simulink model "Regelstrecke_lineare_Zustandsrueckfuehrung"  (R2025a)
settings: Solver=ode15s  StartTime=0.0  StopTime=10
InitFcn:
  | % Definition der Konstanten
  | k  = 1.380649e-23;
  | e  = 1.602176634e-19;
  | T0 = 273.15; % absoluter Nullpunkt in K
  | T_C = 25; % Temperatur in °C
  | UT = k * (T0 + T_C) / e;
  | IS = 1e-8;
  | R  = 1e3;
  | L  = 100e-3;
  | C1 = 100e-9;
  | C2 = 1e-6;
  | 
  | % Werte der Stellgrößen
  | I0 = 10e-3;
  | U0 = 12;
  | 
  | % Berechnung von U2 in der GGL
  | U2_bar = -UT*log(1e8*I0);
  | 
  | % Vorgabe der Eigenwerte
  | eigenvalues = [-200-200i; -200+200i; -500];
  | 
  | % Jacobi-Matrizen an der GGL
  | A = [0 IS/(C1*UT)*exp(-U2_bar/UT) 1/C1;
  |      0 0 1/C2;
  |     -1/L -1/L -R/L];
  | B = [0, 0;
  |      0, -1/C2;
  |      1/L, 0];
  | 
  | % Berechnung der Reglermatrix G
  | G = place(A,B,eigenvalues);
settings Model: Creator=richa  LastModifiedBy=richa

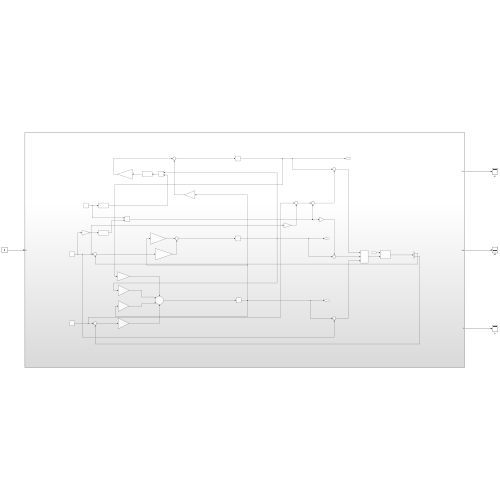
[thumbnail: Simulink's stored preview of the top-level diagram]
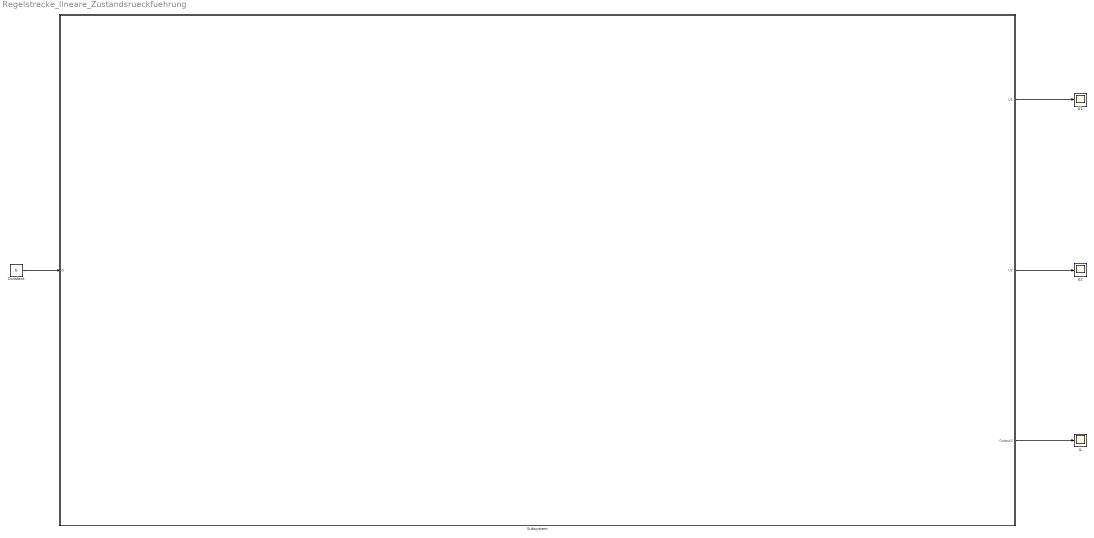
== system Regelstrecke_lineare_Zustandsrueckfuehrung ==
  Constant : Constant  Value=G
  IL : Scope
      settings: ActiveDisplayYMinimum=-0.00074885563020971307  ActiveDisplayYMaximum=0.01042148739337458  DataLoggingVariableName=ScopeData2
  Subsystem : Subsystem
  U1 : Scope
      settings: ActiveDisplayYMinimum=-2.2337880911917134  ActiveDisplayYMaximum=11.108858915218935
  U2 : Scope
      settings: ActiveDisplayYMinimum=-0.762626588701693  ActiveDisplayYMaximum=2.7915785481526711
  wires:
  Subsystem/1(U1) -> U1/1
  Subsystem/2(U2) -> U2/1
  Subsystem/3(Output2) -> IL/1
  Constant/1 -> Subsystem/1("G ")

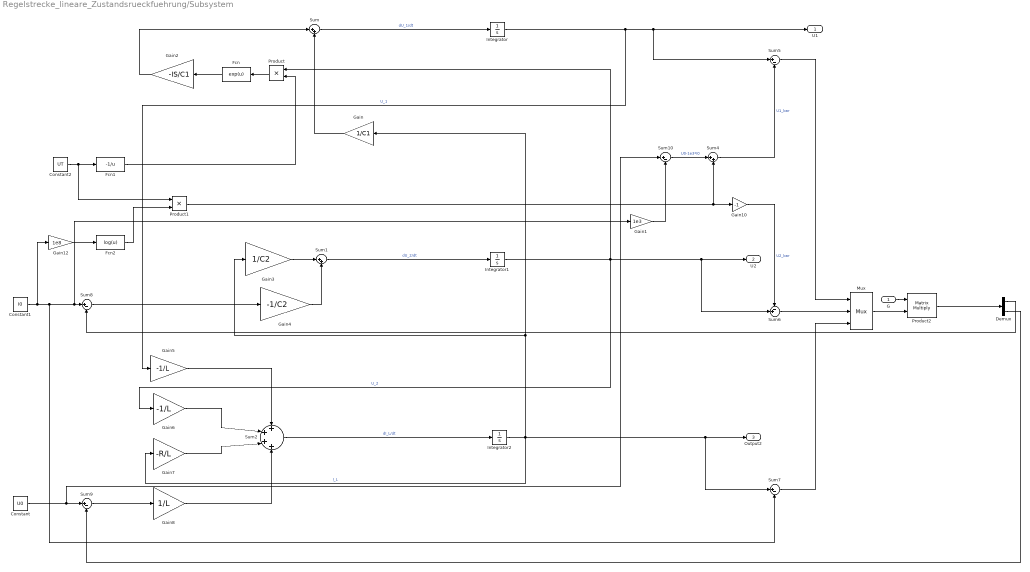
== system Regelstrecke_lineare_Zustandsrueckfuehrung/Subsystem ==
  "G " : Inport
  Constant : Constant  Value=U0
  Constant1 : Constant  Value=I0
  Constant2 : Constant  Value=UT
  Demux : Demux  Outputs=2
  Fcn : Fcn  Expr=exp(u)
  Fcn1 : Fcn  Expr=-1/u
  Fcn2 : Fcn  Expr=log(u)
  Gain : Gain  Gain=1/C1
  Gain1 : Gain  Gain=1e3
  Gain10 : Gain  Gain=-1
  Gain12 : Gain  Gain=1e8
  Gain2 : Gain  Gain=-IS/C1
  Gain3 : Gain  Gain=1/C2
  Gain4 : Gain  Gain=-1/C2
  Gain5 : Gain  Gain=-1/L
  Gain6 : Gain  Gain=-1/L
  Gain7 : Gain  Gain=-R/L
  Gain8 : Gain  Gain=1/L
  Integrator : Integrator
  Integrator1 : Integrator
  Integrator2 : Integrator
  Mux : Mux  Inputs=3
  Product : Product
  Product1 : Product
  Product2 : Product  Multiplication=Matrix(*)
  Sum : Sum  Inputs=|++
  Sum1 : Sum  Inputs=|++
  Sum{5,7..10} (5 alike) : Sum  Inputs=|+-
  Sum2 : Sum  Inputs=++++
  Sum4 : Sum  Inputs=|++
  Sum6 : Sum  Inputs=-+|
  U1 : Outport
  U2 : Outport  Port=2
  Output2 : Outport  Port=3
  wires:
  Integrator/1 -> U1/1, Sum5/1, Gain5/1  "U_1"
  Integrator2/1 -> Output2/1, Sum7/1, Gain7/1, Gain/1, Gain3/1  "I_L"
  Gain4/1 -> Sum1/2
  Product/1 -> Fcn/1
  Constant2/1 -> Product1/1, Fcn1/1
  Gain/1 -> Sum/2
  Integrator1/1 -> U2/1, Sum6/2, Product/1, Gain6/1  "U_2"
  Gain10/1 -> Sum6/1  "U2_bar"
  Gain8/1 -> Sum2/4
  Gain3/1 -> Sum1/1
  Constant1/1 -> Gain12/1, Gain1/1, Sum8/1, Sum7/2
  Sum/1 -> Integrator/1  "dU_1/dt"
  Sum5/1 -> Mux/1
  Fcn1/1 -> Product/2
  Sum6/1 -> Mux/2
  Demux/2 -> Sum9/2
  Gain2/1 -> Sum/1
  Gain5/1 -> Sum2/1
  Sum8/1 -> Gain4/1
  Sum2/1 -> Integrator2/1  "dI_L/dt"
  Gain6/1 -> Sum2/2
  Sum4/1 -> Sum5/2  "U1_bar"
  Mux/1 -> Product2/2
  Sum10/1 -> Sum4/1  "U0-1e3*I0"
  Sum9/1 -> Gain8/1
  Product1/1 -> Gain10/1, Sum4/2
  Demux/1 -> Sum8/2
  Gain7/1 -> Sum2/3
  Fcn/1 -> Gain2/1
  Sum1/1 -> Integrator1/1  "dU_2/dt"
  Sum7/1 -> Mux/3
  Gain12/1 -> Fcn2/1
  Fcn2/1 -> Product1/2
  Gain1/1 -> Sum10/2
  Product2/1 -> Demux/1
  "G "/1 -> Product2/1
  Constant/1 -> Sum9/1, Sum10/1
